simulink model "COMPONENT_MDL_Lag_QUAD_and_PEND_with_spin_rotors"  (R2020b)
settings: Solver=ode23t  StartTime=0.0  StopTime=200  FixedStep=0.001  RelTol=1e-5  EnableMultiTasking=on
undefined symbols (not defined in the file): P_pend, P_rot, P_veh_no_props
(part 6 of 10)

== matlab function COMPONENT_MDL_Lag_QUAD_and_PEND_with_spin_rotors/bh_6DOF_and_pend/Vg_to_Vb/bRg1 ==
  data: phi input; bRg output; theta input; psi input
function bRg = bRg(phi,theta,psi)
%#codegen

%    This function was generated by the Symbolic Math Toolbox version 7.2.
%    28-Aug-2017 09:46:25

bRg = reshape([cos(phi).*cos(theta),-cos(psi).*sin(phi)+cos(phi).*sin(psi).*sin(theta),sin(phi).*sin(psi)+cos(phi).*cos(psi).*sin(theta),cos(theta).*sin(phi),cos(phi).*cos(psi)+sin(phi).*sin(psi).*sin(theta),-cos(phi).*sin(psi)+cos(psi).*sin(phi).*sin(theta),-sin(theta),cos(theta).*sin(psi),cos(psi).*cos(theta)],[3,3]);

== matlab function COMPONENT_MDL_Lag_QUAD_and_PEND_with_spin_rotors/bh_6DOF_and_pend/bRg ==
  data: phi input; bRg output; theta input; psi input
function bRg = bRg(phi,theta,psi)
%#codegen

%    This function was generated by the Symbolic Math Toolbox version 7.2.
%    28-Aug-2017 08:55:21

bRg = reshape([cos(phi).*cos(theta),-cos(psi).*sin(phi)+cos(phi).*sin(psi).*sin(theta),sin(phi).*sin(psi)+cos(phi).*cos(psi).*sin(theta),cos(theta).*sin(phi),cos(phi).*cos(psi)+sin(phi).*sin(psi).*sin(theta),-cos(phi).*sin(psi)+cos(psi).*sin(phi).*sin(theta),-sin(theta),cos(theta).*sin(psi),cos(psi).*cos(theta)],[3,3]);

== matlab function COMPONENT_MDL_Lag_QUAD_and_PEND_with_spin_rotors/bh_6DOF_and_pend/calc_wb/calc_w_from_eul_rates ==
  data: THE_Theta input; wb output; THE_Psi input; THE_PhiD input; THE_ThetaD input; THE_PsiD input
function wb = calc_w_from_eul_rates(THE_Theta,THE_Psi,THE_PhiD,THE_ThetaD,THE_PsiD)
%#codegen

%    This function was generated by the Symbolic Math Toolbox version 7.2.
%    28-Aug-2017 10:05:21

wb = [THE_PsiD-THE_PhiD.*sin(THE_Theta);THE_ThetaD.*cos(THE_Psi)+THE_PhiD.*cos(THE_Theta).*sin(THE_Psi);-THE_ThetaD.*sin(THE_Psi)+THE_PhiD.*cos(THE_Psi).*cos(THE_Theta)];

== matlab function COMPONENT_MDL_Lag_QUAD_and_PEND_with_spin_rotors/bh_6DOF_and_pend/integrate/bRg ==
  data: phi input; bRg output; theta input; psi input
function bRg = bRg(phi,theta,psi)
%#codegen

%    This function was generated by the Symbolic Math Toolbox version 7.2.
%    28-Aug-2017 10:05:16

bRg = reshape([cos(phi).*cos(theta),-cos(psi).*sin(phi)+cos(phi).*sin(psi).*sin(theta),sin(phi).*sin(psi)+cos(phi).*cos(psi).*sin(theta),cos(theta).*sin(phi),cos(phi).*cos(psi)+sin(phi).*sin(psi).*sin(theta),-cos(phi).*sin(psi)+cos(psi).*sin(phi).*sin(theta),-sin(theta),cos(theta).*sin(psi),cos(psi).*cos(theta)],[3,3]);

== matlab function COMPONENT_MDL_Lag_QUAD_and_PEND_with_spin_rotors/bh_6DOF_and_pend/create pend_BUS/MATLAB Function ==
  data: phi input; wb output; theta input; psi input; phi_dot input; theta_dot input; psi_dot input
function wb = fcn(phi,theta,psi, phi_dot, theta_dot, psi_dot)

A = [ ...
             -sin(theta),         0, 1;
        cos(theta)*sin(psi),  cos(psi), 0;
        cos(psi)*cos(theta), -sin(psi), 0;  ];


x = [    phi_dot;
       theta_dot; 
         psi_dot;  ];  
    


wb = A * x;

== matlab function COMPONENT_MDL_Lag_QUAD_and_PEND_with_spin_rotors/bh_6DOF_and_pend/integrate/calc_eul_rates_from_w ==
  data: THE_Theta input; edot output; THE_Psi input; p input; q input; r input
function edot = calc_eul_rates_from_w(THE_Theta,THE_Psi,p,q,r)
%#codegen

%    This function was generated by the Symbolic Math Toolbox version 7.2.
%    28-Aug-2017 10:05:22

edot = [(r.*cos(THE_Psi)+q.*sin(THE_Psi))./cos(THE_Theta);q.*cos(THE_Psi)-r.*sin(THE_Psi);(p.*cos(THE_Theta)+r.*cos(THE_Psi).*sin(THE_Theta)+q.*sin(THE_Psi).*sin(THE_Theta))./cos(THE_Theta)];

== matlab function COMPONENT_MDL_Lag_QUAD_and_PEND_with_spin_rotors/bh_6DOF_and_pend/create pend_BUS/bRg ==
  data: phi input; bRg output; theta input; psi input
function bRg = bRg(phi,theta,psi)
%#codegen

%    This function was generated by the Symbolic Math Toolbox version 7.2.
%    28-Aug-2017 08:55:21

bRg = reshape([cos(phi).*cos(theta),-cos(psi).*sin(phi)+cos(phi).*sin(psi).*sin(theta),sin(phi).*sin(psi)+cos(phi).*cos(psi).*sin(theta),cos(theta).*sin(phi),cos(phi).*cos(psi)+sin(phi).*sin(psi).*sin(theta),-cos(phi).*sin(psi)+cos(psi).*sin(phi).*sin(theta),-sin(theta),cos(theta).*sin(psi),cos(psi).*cos(theta)],[3,3]);

== matlab function COMPONENT_MDL_Lag_QUAD_and_PEND_with_spin_rotors/bh_6DOF_and_pend/solve_for_qDD/MATLAB Function ==
  data: M input; the_cond output
function the_cond = COND(M)
%#codegen

the_cond = cond(M);

end

== matlab function COMPONENT_MDL_Lag_QUAD_and_PEND_with_spin_rotors/bh_6DOF_and_pend/MATLAB Function ==
  data: I input; Ixx output; Ixy output; Ixz output; Iyy output; Iyz output; Izz output
function [Ixx, Ixy, Ixz, Iyy, Iyz, Izz] = fcn(I)

Ixx = I(1,1); 
Ixy = I(1,2); 
Ixz = I(1,3); 
Iyy = I(2,2); 
Iyz = I(2,3); 
Izz = I(3,3);

end
